simulink model "point7"  (R2018a)
settings: Solver=VariableStepAuto  StartTime=0  StopTime=10  RelTol=1e-3
settings Model: Creator=Yan Tszyafen  LastModifiedBy=Yan Tszyafen

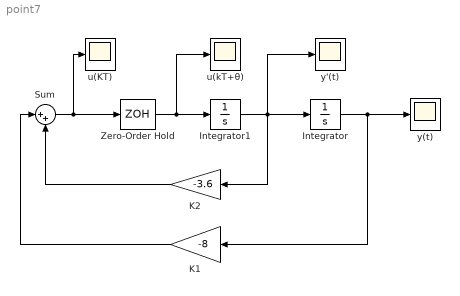
== system point7 ==
  Integrator : Integrator  InitialCondition=1
  Integrator1 : Integrator
  K1 : Gain  Gain=-8
  K2 : Gain  Gain=-3.6
  Sum : Sum  Inputs=|++
  Zero-Order Hold : ZeroOrderHold  SampleTime=0.1
  u(KT) : Scope
  u(kT+θ) : Scope
  y'(t) : Scope
  y(t) : Scope
  wires:
  Sum/1 -> u(KT)/1, Zero-Order Hold/1
  Zero-Order Hold/1 -> u(kT+θ)/1, Integrator1/1
  Integrator1/1 -> y'(t)/1, K2/1, Integrator/1
  K2/1 -> Sum/2
  K1/1 -> Sum/1
  Integrator/1 -> y(t)/1, K1/1
